simulink model "sim_new_traj_only_att_ctrl"  (R2020a)
settings: Solver=ode4  StartTime=0.0  StopTime=30.0  FixedStep=0.01  RelTol=1e-3
values from neighbouring files (symbols this model uses):
  beta_Phi_1 = pp0 * cal_frac_squ( 3, p_p0_plus_1, q_p0_plus_1 )                          * cal_frac_squ( eps_s_bar / pi, p_p0_min_2, q_p0_min_2 )                          / ( 2 * ( 2 * pp0 - 1 ) * tanh( gamma0 * ( eps_s_bar / pi ) / 2 ) )                          - ( cal_frac_squ( 3, p_p0_plus_1, q_p0_plus_1 ) * gamma0 / ( 4 * ( 2 * pp0 -1 ) ) )                          * cal_frac_squ( eps_s_bar / pi, p_p0_min_ ...(+136 chars)    [init_new_traj_only_att_ctrl.m]
  beta_Phi_2 = ( 1 - pp0 ) * cal_frac_squ( 3, p_p0_plus_1, q_p0_plus_1 )                          / ( 2 * ( 1 - 2 * pp0 ) * cal_frac_squ( eps_s_bar / pi, p_p0_0, q_p0_0 ) * tanh( gamma0 * ( eps_s_bar / pi ) / 2 ) )                          - ( cal_frac_squ( 3, p_p0_plus_1, q_p0_plus_1 ) * gamma0 / ( 4 * ( 1 - 2 * pp0 ) ) )                          * cal_frac_squ( eps_s_bar / pi, p_1_min_p0, q_1_min_p0 )          ...(+112 chars)    [init_new_traj_only_att_ctrl.m]
  c1_diff_sigma_bar_w = diag([12; 12; 12])    [init_new_traj_only_att_ctrl.m]
  c1_diff_ui = diag([25; 30; 20])    [init_new_traj_only_att_ctrl.m]
  c2_diff_sigma_bar_w = diag([12; 12; 12])    [init_new_traj_only_att_ctrl.m]
  c2_diff_ui = diag([50; 50; 10])    [init_new_traj_only_att_ctrl.m]
  c3_diff_sigma_bar_w = diag([15; 15; 15])    [init_new_traj_only_att_ctrl.m]
  c3_diff_ui = diag([15; 15; 10])    [init_new_traj_only_att_ctrl.m]
  c_w_1 = diag( [20; 15; 15] )    [init_new_traj_only_att_ctrl.m]
  c_w_2 = diag( [20; 15; 15] )    [init_new_traj_only_att_ctrl.m]
  c_w_3 = diag( [2; 2; 2] )    [init_new_traj_only_att_ctrl.m]
  cS0 = diag( [4.5; 4.5; 4.5] )    [init_new_traj_only_att_ctrl.m]
  dw_aa_t = 0.2 * ones(3, 5) + ( 1.0 - 0.2 ) * rand(3, 5)    [init_new_traj_only_att_ctrl.m]
  dw_ff_t = [ 0.4 * ones(1, 5) + ( 1.0 - 0.4 ) * rand(1, 5);                      0.4 * ones(1, 5) + ( 1.0 - 0.4 ) * rand(1, 5);                      0.2 * ones(1, 5) + ( 0.6 - 0.2 ) * rand(1, 5) ]    [init_new_traj_only_att_ctrl.m]
  dw_phi_t = ( - pi / 2 ) * ones(3, 5) + ( pi / 2 - ( - pi / 2 ) ) * rand(3, 5)    [init_new_traj_only_att_ctrl.m]
  dwci_init = zeros(3,5)    [init_new_traj_only_att_ctrl.m]
  eps_s_bar_div_pi = eps_s_bar / pi    (= 0.03)    [init_new_traj_only_att_ctrl.m]
  gamma0 = 20    [init_new_traj_only_att_ctrl.m]
  h1w = diag([20.0; 20.0; 20.0])    [init_new_traj_only_att_ctrl.m]
  h2w = diag([30.0; 35.0; 35.0])    [init_new_traj_only_att_ctrl.m]
  h3w = diag([30.0; 25.0; 30.0])    [init_new_traj_only_att_ctrl.m]
  Ji = zeros(3,3,NF)    [init_new_traj_only_att_ctrl.m]
  k_J_0 = diag( [1; 1; 1] )    [init_new_traj_only_att_ctrl.m]
  Lamd_diff_sigma_bar_w = 0.8    [init_new_traj_only_att_ctrl.m]
  Lamd_diff_ui = 0.8    [init_new_traj_only_att_ctrl.m]
  mu_c_theta = 100    [init_new_traj_only_att_ctrl.m]
  mu_d_w = 100    [init_new_traj_only_att_ctrl.m]
  pos0 = zeros(3, 1)    [init_new_traj_only_att_ctrl.m]
  pp0 = 8 / 11    (= 0.727272727273)    [init_new_traj_only_att_ctrl.m]
  PZ0 = P0(3)    [init_new_traj_only_att_ctrl.m]
  PZ1 = 10    [init_new_traj_only_att_ctrl.m]
  Qci_init = repmat([1;0;0;0],1,NF)    [init_new_traj_only_att_ctrl.m]
  R0 = 4    [init_new_traj_only_att_ctrl.m]
  R1 = 8    [init_new_traj_only_att_ctrl.m]
  Rci_init = zeros(3,3,NF)    [init_new_traj_only_att_ctrl.m]
  Ri_init = zeros(3,3,NF)    [init_new_traj_only_att_ctrl.m]
  Rx2 = 10    [init_new_traj_only_att_ctrl.m]
  Ry2 = 6    [init_new_traj_only_att_ctrl.m]
  Rz2 = 4    [init_new_traj_only_att_ctrl.m]
  T0 = 0    [init_new_traj_only_att_ctrl.m]
  T1 = tseq1    (= 10)    [init_new_traj_only_att_ctrl.m]
  T2 = tseq1 + tseq12 + tseq2    (= 30)    [init_new_traj_only_att_ctrl.m]
  thr_p_plus_1 = cal_frac_squ( 3, p_p0_plus_1, q_p0_plus_1 )    [init_new_traj_only_att_ctrl.m]
  ui_init = zeros(3,NF)    [init_new_traj_only_att_ctrl.m]
  vel0 = zeros(3, 1)    [init_new_traj_only_att_ctrl.m]
  wci_init = zeros(3,5)    [init_new_traj_only_att_ctrl.m]
  zeta_diff_sigma_bar_w = 0.3    [init_new_traj_only_att_ctrl.m]
  zeta_diff_ui = 0.05    [init_new_traj_only_att_ctrl.m]
undefined symbols (not defined in the file or in its folder): cal_frac_squ, p_2_p0, p_alfaw1, p_alfaw2, p_beta_w_1, p_beta_w_2, p_p0_min_1, p_p0_plus_1, q_2_p0, q_alfaw1, q_alfaw2, q_beta_w_1, q_beta_w_2, q_p0_min_1, q_p0_plus_1, Qei_init, Qi_init, Rei_init, V_Phi_Rei_init, wei_init, wi_init
(part 4 of 5)

== matlab function sim_new_traj_only_att_ctrl/cal wci dwci agent 5 ==
  data: ui_vec input; wci output; duihat_vec input; d2uihat_vec input; Rci_mat input; dwci output
function [wci, dwci] = fcn(ui_vec, duihat_vec, d2uihat_vec, Rci_mat)
%%%% 计算姿态角速率指令及其导数

iiuav = 5;
ui = ui_vec(:,iiuav);
duihat = duihat_vec(:,iiuav);
d2uihat = d2uihat_vec(:,iiuav);
Rci = Rci_mat(:,:,iiuav);

ee1 = [1;0;0];
ee2 = [0;1;0];
ee3 = [0;0;1];
RciE3 = ui / norm(ui,2);
PiMat = eye(3,3) - ee3*(ee3');
dRciE3 = (1 / norm(ui,2))*Rci*PiMat*(Rci')*duihat;
Themat = [-RciE3(2)/(1+RciE3(3)),         -RciE3(1)/(1+RciE3(3)),       (RciE3(1)*RciE3(2))/((1+RciE3(3))^2); ...
                   2*RciE3(1)/(1+RciE3(3)),                0,                               1 - (RciE3(1)^2)/((1+RciE3(3))^2); ...
                               0                                       -1                                                        0                                   ];
wcxe3 = (1 / norm(ui,2))*PiMat*(Rci')*duihat;
wcxe2 = (1 / norm(ui,2))*(Rci')*Themat*Rci*PiMat*(Rci')*duihat;
wci = [-wcxe3(2); wcxe3(1); -wcxe2(1)];

TempMat1 = [0,                           -1/(1+RciE3(3)),                   (RciE3(2))/((1+RciE3(3))^2); ...
                       2/(1+RciE3(3)),                0,                               (-2*RciE3(1))/((1+RciE3(3))^2); ...
                       0,                                     0,                                                   0                             ];
TempMat2 = [-1/(1+RciE3(3)),              0,                               (RciE3(1))/((1+RciE3(3))^2); ...
                       0,                                     0,                                                   0                      ; ...
                       0,                                     0,                                                   0                             ];
TempMat3 = [(RciE3(2))/((1+RciE3(3))^2),                 (RciE3(1))/((1+RciE3(3))^2),       (-2*RciE3(1)*RciE3(2))/((1+RciE3(3))^3); ...
                       (-2*RciE3(1))/((1+RciE3(3))^2),                             0,                               (2*(RciE3(1)^2))/((1+RciE3(3))^3); ...
                        0,                                                                          0,                                                   0                             ];
dTheMat = TempMat1*dRciE3*(ee1') + TempMat2*dRciE3*(ee2') + TempMat3*dRciE3*(ee3');
wcix = cal_askew_mat(wci);
dRciT = -wcix*(Rci');
dwcxe3 = (1 / norm(ui,2))*PiMat*(dRciT*duihat+(Rci')*(d2uihat-(((ui')*duihat)/(norm(ui,2)^2))*duihat));
dwcxe2 = (1 / norm(ui,2))*((dRciT*Themat+(Rci')*dTheMat) ...
                *(Rci*PiMat*(Rci'))*duihat + (Rci')*Themat*(Rci*PiMat*(Rci'))*(d2uihat-(((ui')*duihat)/(norm(ui,2)^2))*duihat));
dwci = [-dwcxe3(2);  dwcxe3(1);  -dwcxe2(1)];

== matlab function sim_new_traj_only_att_ctrl/cal wei agent 1 ==
  data: wi_vec input; wei_1 output; Rei_vec input; wci_vec input
function wei_1 = fcn(wi_vec, Rei_vec, wci_vec)
%%%% 更新姿态角速率误差
iiuav = 1;
wei_1 = wi_vec(:,iiuav) - (Rei_vec(:,:,iiuav)') * wci_vec(:,iiuav);

end

== matlab function sim_new_traj_only_att_ctrl/cal wei agent 2 ==
  data: wi_vec input; wei_2 output; Rei_vec input; wci_vec input
function wei_2 = fcn(wi_vec, Rei_vec, wci_vec)
%%%% 更新姿态角速率误差
iiuav = 2;
wei_2 = wi_vec(:,iiuav) - (Rei_vec(:,:,iiuav)') * wci_vec(:,iiuav);

end

== matlab function sim_new_traj_only_att_ctrl/cal wei agent 3 ==
  data: wi_vec input; wei_3 output; Rei_vec input; wci_vec input
function wei_3 = fcn(wi_vec, Rei_vec, wci_vec)
%%%% 更新姿态角速率误差
iiuav = 3;
wei_3 = wi_vec(:,iiuav) - (Rei_vec(:,:,iiuav)') * wci_vec(:,iiuav);

end

== matlab function sim_new_traj_only_att_ctrl/cal wei agent 4 ==
  data: wi_vec input; wei_4 output; Rei_vec input; wci_vec input
function wei_4 = fcn(wi_vec, Rei_vec, wci_vec)
%%%% 更新姿态角速率误差
iiuav = 4;
wei_4 = wi_vec(:,iiuav) - (Rei_vec(:,:,iiuav)') * wci_vec(:,iiuav);

end

== matlab function sim_new_traj_only_att_ctrl/cal wei agent 5 ==
  data: wi_vec input; wei_5 output; Rei_vec input; wci_vec input
function wei_5 = fcn(wi_vec, Rei_vec, wci_vec)
%%%% 更新姿态角速率误差
iiuav = 5;
wei_5 = wi_vec(:,iiuav) - (Rei_vec(:,:,iiuav)') * wci_vec(:,iiuav);

end

== matlab function sim_new_traj_only_att_ctrl/choose ksi_est_err 41 ==
  data: x input; y output
function y = fcn(x)
iiuav = 1;
y = x(:,iiuav);

== matlab function sim_new_traj_only_att_ctrl/choose ksi_est_err 42 ==
  data: x input; y output
function y = fcn(x)
iiuav = 5;
y = x(:,iiuav);

== matlab function sim_new_traj_only_att_ctrl/choose ksi_est_err 43 ==
  data: x input; y output
function y = fcn(x)
iiuav = 1;
y = x(:,iiuav);

== matlab function sim_new_traj_only_att_ctrl/choose ksi_est_err 44 ==
  data: x input; y output
function y = fcn(x)
iiuav = 1;
y = x(:,iiuav);

== matlab function sim_new_traj_only_att_ctrl/choose ksi_est_err 45 ==
  data: x input; y output
function y = fcn(x)
iiuav = 2;
y = x(:,iiuav);

== matlab function sim_new_traj_only_att_ctrl/choose ksi_est_err 46 ==
  data: x input; y output
function y = fcn(x)
iiuav = 2;
y = x(:,iiuav);

== matlab function sim_new_traj_only_att_ctrl/choose ksi_est_err 47 ==
  data: x input; y output
function y = fcn(x)
iiuav = 3;
y = x(:,iiuav);

== matlab function sim_new_traj_only_att_ctrl/choose ksi_est_err 48 ==
  data: x input; y output
function y = fcn(x)
iiuav = 3;
y = x(:,iiuav);

== matlab function sim_new_traj_only_att_ctrl/choose ksi_est_err 49 ==
  data: x input; y output
function y = fcn(x)
iiuav = 4;
y = x(:,iiuav);

== matlab function sim_new_traj_only_att_ctrl/cal Fi_S agent 4 ==
  data: cS0 input; Ji input; wi_vec input; wci_vec input; wei_vec input; Fi_S_4 output; dwci_vec input; Rei_vec input; Phi_bar_psi_e_vec input
function Fi_S_4 = fcn(cS0, Ji, wi_vec, wci_vec, wei_vec, dwci_vec, Rei_vec, Phi_bar_psi_e_vec)
%%%% 计算补偿项
iiuav = 4;
Fi_S_4 = -cal_askew_mat( wi_vec(:,iiuav) ) * Ji(:,:,iiuav) * wi_vec(:,iiuav) ...
                + Ji(:,:,iiuav) * cal_askew_mat( wei_vec(:,iiuav) ) * ( Rei_vec(:,:,iiuav)' ) * wci_vec(:,iiuav) ...
                - Ji(:,:,iiuav) * ( Rei_vec(:,:,iiuav)' ) * dwci_vec(:,iiuav) ...
                + cS0 * Ji(:,:,iiuav) * Phi_bar_psi_e_vec(:,iiuav);

== matlab function sim_new_traj_only_att_ctrl/choose ksi_est_err 50 ==
  data: x input; y output
function y = fcn(x)
iiuav = 4;
y = x(:,iiuav);

== matlab function sim_new_traj_only_att_ctrl/choose ksi_est_err 51 ==
  data: x input; y output
function y = fcn(x)
iiuav = 5;
y = x(:,iiuav);

== matlab function sim_new_traj_only_att_ctrl/choose ksi_est_err 52 ==
  data: x input; y output
function y = fcn(x)
iiuav = 1;
y = x(:,iiuav);

== matlab function sim_new_traj_only_att_ctrl/choose ksi_est_err 53 ==
  data: x input; y output
function y = fcn(x)
iiuav = 5;
y = x(:,iiuav);

== matlab function sim_new_traj_only_att_ctrl/choose ksi_est_err 54 ==
  data: x input; y output
function y = fcn(x)
iiuav = 1;
y = x(:,iiuav);

== matlab function sim_new_traj_only_att_ctrl/choose ksi_est_err 55 ==
  data: x input; y output
function y = fcn(x)
iiuav = 2;
y = x(:,iiuav);

== matlab function sim_new_traj_only_att_ctrl/choose ksi_est_err 56 ==
  data: x input; y output
function y = fcn(x)
iiuav = 3;
y = x(:,iiuav);

== matlab function sim_new_traj_only_att_ctrl/choose ksi_est_err 57 ==
  data: x input; y output
function y = fcn(x)
iiuav = 4;
y = x(:,iiuav);

== matlab function sim_new_traj_only_att_ctrl/choose ksi_est_err 58 ==
  data: x input; y output
function y = fcn(x)
iiuav = 5;
y = x(:,iiuav);

== matlab function sim_new_traj_only_att_ctrl/choose ksi_est_err 59 ==
  data: x input; y output
function y = fcn(x)
iiuav = 1;
y = x(:,iiuav);

== matlab function sim_new_traj_only_att_ctrl/choose ksi_est_err 60 ==
  data: x input; y output
function y = fcn(x)
iiuav = 1;
y = x(:,iiuav);

== matlab function sim_new_traj_only_att_ctrl/choose ksi_est_err 61 ==
  data: x input; y output
function y = fcn(x)
iiuav = 2;
y = x(:,iiuav);

== matlab function sim_new_traj_only_att_ctrl/choose ksi_est_err 62 ==
  data: x input; y output
function y = fcn(x)
iiuav = 2;
y = x(:,iiuav);

== matlab function sim_new_traj_only_att_ctrl/choose ksi_est_err 63 ==
  data: x input; y output
function y = fcn(x)
iiuav = 2;
y = x(:,iiuav);

== matlab function sim_new_traj_only_att_ctrl/choose ksi_est_err 64 ==
  data: x input; y output
function y = fcn(x)
iiuav = 3;
y = x(:,iiuav);

== matlab function sim_new_traj_only_att_ctrl/choose ksi_est_err 65 ==
  data: x input; y output
function y = fcn(x)
iiuav = 3;
y = x(:,iiuav);

== matlab function sim_new_traj_only_att_ctrl/choose ksi_est_err 66 ==
  data: x input; y output
function y = fcn(x)
iiuav = 4;
y = x(:,iiuav);

== matlab function sim_new_traj_only_att_ctrl/choose ksi_est_err 67 ==
  data: x input; y output
function y = fcn(x)
iiuav = 4;
y = x(:,iiuav);

== matlab function sim_new_traj_only_att_ctrl/choose ksi_est_err 68 ==
  data: x input; y output
function y = fcn(x)
iiuav = 5;
y = x(:,iiuav);

== matlab function sim_new_traj_only_att_ctrl/choose ksi_est_err 69 ==
  data: x input; y output
function y = fcn(x)
iiuav = 5;
y = x(:,iiuav);

== matlab function sim_new_traj_only_att_ctrl/cal Fi_S agent 5 ==
  data: cS0 input; Ji input; wi_vec input; wci_vec input; wei_vec input; Fi_S_5 output; dwci_vec input; Rei_vec input; Phi_bar_psi_e_vec input
function Fi_S_5 = fcn(cS0, Ji, wi_vec, wci_vec, wei_vec, dwci_vec, Rei_vec, Phi_bar_psi_e_vec)
%%%% 计算补偿项
iiuav = 5;
Fi_S_5 = -cal_askew_mat( wi_vec(:,iiuav) ) * Ji(:,:,iiuav) * wi_vec(:,iiuav) ...
                + Ji(:,:,iiuav) * cal_askew_mat( wei_vec(:,iiuav) ) * ( Rei_vec(:,:,iiuav)' ) * wci_vec(:,iiuav) ...
                - Ji(:,:,iiuav) * ( Rei_vec(:,:,iiuav)' ) * dwci_vec(:,iiuav) ...
                + cS0 * Ji(:,:,iiuav) * Phi_bar_psi_e_vec(:,iiuav);

== matlab function sim_new_traj_only_att_ctrl/choose ksi_est_err 70 ==
  data: x input; y output
function y = fcn(x)
iiuav = 2;
y = x(:,iiuav);

== matlab function sim_new_traj_only_att_ctrl/choose ksi_est_err 71 ==
  data: x input; y output
function y = fcn(x)
iiuav = 3;
y = x(:,iiuav);

== matlab function sim_new_traj_only_att_ctrl/choose ksi_est_err 72 ==
  data: x input; y output
function y = fcn(x)
iiuav = 3;
y = x(:,iiuav);

== matlab function sim_new_traj_only_att_ctrl/choose ksi_est_err 73 ==
  data: x input; y output
function y = fcn(x)
iiuav = 4;
y = x(:,iiuav);

== matlab function sim_new_traj_only_att_ctrl/choose ksi_est_err 74 ==
  data: x input; y output
function y = fcn(x)
iiuav = 4;
y = x(:,iiuav);

== matlab function sim_new_traj_only_att_ctrl/choose ksi_est_err 75 ==
  data: x input; y output
function y = fcn(x)
iiuav = 5;
y = x(:,iiuav);

== matlab function sim_new_traj_only_att_ctrl/choose ui agent 1 ==
  data: x input; y output
function y = fcn(x)
iiuav = 1;
y = x(:,iiuav);

== matlab function sim_new_traj_only_att_ctrl/choose ui agent 2 ==
  data: x input; y output
function y = fcn(x)
iiuav = 2;
y = x(:,iiuav);

== matlab function sim_new_traj_only_att_ctrl/choose ui agent 3 ==
  data: x input; y output
function y = fcn(x)
iiuav = 3;
y = x(:,iiuav);

== matlab function sim_new_traj_only_att_ctrl/choose ui agent 4 ==
  data: x input; y output
function y = fcn(x)
iiuav = 4;
y = x(:,iiuav);

== matlab function sim_new_traj_only_att_ctrl/choose ui agent 5 ==
  data: x input; y output
function y = fcn(x)
iiuav = 5;
y = x(:,iiuav);

== matlab function sim_new_traj_only_att_ctrl/combine Fi_S ==
  data: Fi_S_1 input; Fi_S_2 input; Fi_S_3 input; Fi_S_4 input; Fi_S_5 input; Fi_S_vec output
function Fi_S_vec  = fcn(Fi_S_1, Fi_S_2, Fi_S_3, Fi_S_4, Fi_S_5)
%%%% 合并补偿项
Fi_S_vec = zeros(3,5);
Fi_S_vec(:,1) = Fi_S_1(:);
Fi_S_vec(:,2) = Fi_S_2(:);
Fi_S_vec(:,3) = Fi_S_3(:);
Fi_S_vec(:,4) = Fi_S_4(:);
Fi_S_vec(:,5) = Fi_S_5(:);

== matlab function sim_new_traj_only_att_ctrl/combine Phi_bar_psi_e ==
  data: Phi_bar_psi_e_node_1 input; Phi_bar_psi_e_node_2 input; Phi_bar_psi_e_node_3 input; Phi_bar_psi_e_node_4 input; Phi_bar_psi_e_node_5 input; Phi_bar_psi_e_vec output
function Phi_bar_psi_e_vec  = fcn(Phi_bar_psi_e_node_1, Phi_bar_psi_e_node_2, Phi_bar_psi_e_node_3, ...
                                                                Phi_bar_psi_e_node_4, Phi_bar_psi_e_node_5)
%%%% 合并姿态误差导数
Phi_bar_psi_e_vec = zeros(3,5);
Phi_bar_psi_e_vec(:,1) = Phi_bar_psi_e_node_1(:);
Phi_bar_psi_e_vec(:,2) = Phi_bar_psi_e_node_2(:);
Phi_bar_psi_e_vec(:,3) = Phi_bar_psi_e_node_3(:);
Phi_bar_psi_e_vec(:,4) = Phi_bar_psi_e_node_4(:);
Phi_bar_psi_e_vec(:,5) = Phi_bar_psi_e_node_5(:);

== matlab function sim_new_traj_only_att_ctrl/combine Phi_psi_e ==
  data: Phi_psi_e_node_1 input; Phi_psi_e_node_2 input; Phi_psi_e_node_3 input; Phi_psi_e_node_4 input; Phi_psi_e_node_5 input; Phi_psi_e_vec output
function Phi_psi_e_vec  = fcn(Phi_psi_e_node_1, Phi_psi_e_node_2, Phi_psi_e_node_3, ...
                                                        Phi_psi_e_node_4, Phi_psi_e_node_5)
%%%% 合并姿态误差项
Phi_psi_e_vec = zeros(3,5);
Phi_psi_e_vec(:,1) = Phi_psi_e_node_1(:);
Phi_psi_e_vec(:,2) = Phi_psi_e_node_2(:);
Phi_psi_e_vec(:,3) = Phi_psi_e_node_3(:);
Phi_psi_e_vec(:,4) = Phi_psi_e_node_4(:);
Phi_psi_e_vec(:,5) = Phi_psi_e_node_5(:);

== matlab function sim_new_traj_only_att_ctrl/combine Qci Rci ==
  data: Qci_1 input; Qci_vec output; Qci_2 input; Qci_3 input; Qci_4 input; Qci_5 input; Rci_1 input; Rci_2 input; Rci_3 input; Rci_4 input; Rci_5 input; Rci_vec output
function [Qci_vec, Rci_vec] = fcn(Qci_1, Qci_2, Qci_3, Qci_4, Qci_5, ...
                                                            Rci_1, Rci_2, Rci_3, Rci_4, Rci_5)
%%%% 合并四元数和姿态旋转矩阵
Qci_vec = zeros(4,5);
Qci_vec(:,1) = Qci_1(:);
Qci_vec(:,2) = Qci_2(:);
Qci_vec(:,3) = Qci_3(:);
Qci_vec(:,4) = Qci_4(:);
Qci_vec(:,5) = Qci_5(:);

Rci_vec = zeros(3,3,5);
Rci_vec(:,:,1) = Rci_1;
Rci_vec(:,:,2) = Rci_2;
Rci_vec(:,:,3) = Rci_3;
Rci_vec(:,:,4) = Rci_4;
Rci_vec(:,:,5) = Rci_5;

== matlab function sim_new_traj_only_att_ctrl/combine Qci Rci1 ==
  data: V_Phi_Rei_1 input; V_Phi_Rei_vec output; V_Phi_Rei_2 input; V_Phi_Rei_3 input; V_Phi_Rei_4 input; V_Phi_Rei_5 input
function V_Phi_Rei_vec = fcn(V_Phi_Rei_1, V_Phi_Rei_2, V_Phi_Rei_3, V_Phi_Rei_4, V_Phi_Rei_5)
%%%% 合并LogSO3空间的辅助姿态误差向量
V_Phi_Rei_vec = [V_Phi_Rei_1(:), V_Phi_Rei_2(:), V_Phi_Rei_3(:), V_Phi_Rei_4(:), V_Phi_Rei_5(:)];

== matlab function sim_new_traj_only_att_ctrl/cal Phi_bar_psi_e agent 1 ==
  data: pp0 input; Phi_bar_psi_e_node_1 output; beta_Phi_1 input; beta_Phi_2 input; thr_p_plus_1 input; gamma0 input; eps_s_bar_div_pi input; wei_vec input; S_bar_vec input; V_Phi_Rei_div_pi_vec input; V_Phi_Rei_squ_p_min_1_vec input; V_Phi_Rei_squ_p_plus_1_vec input; V_Phi_Rei_squ_2p_vec input
function Phi_bar_psi_e_node_1 = fcn(pp0, beta_Phi_1, beta_Phi_2, thr_p_plus_1, gamma0, ...
                                                                    eps_s_bar_div_pi, wei_vec, S_bar_vec, V_Phi_Rei_div_pi_vec, ...
                                                                    V_Phi_Rei_squ_p_min_1_vec, V_Phi_Rei_squ_p_plus_1_vec, V_Phi_Rei_squ_2p_vec)
%%%% 计算姿态误差项
iiuav = 1;
Phi_bar_psi_e_node_1 = zeros(3,1);
for kk = 1:3
    if S_bar_vec(kk, iiuav) == 0
        Phi_bar_psi_e_node_1(kk, 1) = thr_p_plus_1 * ( pp0 + 1 ) * V_Phi_Rei_div_pi_vec(kk, iiuav) ...
                                                                * V_Phi_Rei_squ_p_min_1_vec(kk, iiuav) * wei_vec(kk, iiuav) ...
                                                                / ( 2 * tanh( ( gamma0 / 2 ) * V_Phi_Rei_div_pi_vec(kk, iiuav) ) ) ...
                                                                + ( thr_p_plus_1 * gamma0 / 4 ) * V_Phi_Rei_squ_p_plus_1_vec(kk, iiuav) ...
                                                                * ( ( sech( ( gamma0 / 2 ) * V_Phi_Rei_div_pi_vec(kk, iiuav) ) ...
                                                                / tanh( ( gamma0 / 2 ) * V_Phi_Rei_div_pi_vec(kk, iiuav) ) ) ^ 2 ) * wei_vec(kk, iiuav);
    else
        if abs( V_Phi_Rei_div_pi_vec ) > eps_s_bar_div_pi
            Phi_bar_psi_e_node_1(kk, 1) = thr_p_plus_1 * ( pp0 + 1 ) * V_Phi_Rei_div_pi_vec(kk, iiuav) ...
                                                                    * V_Phi_Rei_squ_p_min_1_vec(kk, iiuav) * wei_vec(kk, iiuav) ...
                                                                    / ( 2 * tanh( ( gamma0 / 2 ) * V_Phi_Rei_div_pi_vec(kk, iiuav) ) ) ...
                                                                    + ( thr_p_plus_1 * gamma0 / 4 ) * V_Phi_Rei_squ_p_plus_1_vec(kk, iiuav) ...
                                                                    * ( ( sech( ( gamma0 / 2 ) * V_Phi_Rei_div_pi_vec(kk, iiuav) ) ...
                                                                    / tanh( ( gamma0 / 2 ) * V_Phi_Rei_div_pi_vec(kk, iiuav) ) ) ^ 2 ) * wei_vec(kk, iiuav);
        else
            Phi_bar_psi_e_node_1(kk, 1) = 2 * beta_Phi_1 * ( ( abs( V_Phi_Rei_div_pi_vec(kk, iiuav) ) ) ^ 2 ) * wei_vec(kk, iiuav) ...
                                                                    + ( 2 * pp0 + 1 ) * beta_Phi_2 * V_Phi_Rei_squ_2p_vec(kk, iiuav) * wei_vec(kk, iiuav);
        end
    end
end

== matlab function sim_new_traj_only_att_ctrl/combine Qi Ri ==
  data: Qi_1 input; Qi_vec output; Qi_2 input; Qi_3 input; Qi_4 input; Qi_5 input; Ri_1 input; Ri_2 input; Ri_3 input; Ri_4 input; Ri_5 input; Ri_vec output
function [Qi_vec, Ri_vec] = fcn(Qi_1, Qi_2, Qi_3, Qi_4, Qi_5, ...
                                                        Ri_1, Ri_2, Ri_3, Ri_4, Ri_5)
%%%% 合并四元数和姿态旋转矩阵
Qi_vec = zeros(4,5);
Qi_vec(:,1) = Qi_1(:);
Qi_vec(:,2) = Qi_2(:);
Qi_vec(:,3) = Qi_3(:);
Qi_vec(:,4) = Qi_4(:);
Qi_vec(:,5) = Qi_5(:);

Ri_vec = zeros(3,3,5);
Ri_vec(:,:,1) = Ri_1;
Ri_vec(:,:,2) = Ri_2;
Ri_vec(:,:,3) = Ri_3;
Ri_vec(:,:,4) = Ri_4;
Ri_vec(:,:,5) = Ri_5;

== matlab function sim_new_traj_only_att_ctrl/combine S_bar ==
  data: S_bar_node_1 input; S_bar_node_2 input; S_bar_node_3 input; S_bar_node_4 input; S_bar_node_5 input; S_bar_vec output
function S_bar_vec  = fcn(S_bar_node_1, S_bar_node_2, S_bar_node_3, ...
                                                S_bar_node_4, S_bar_node_5)
%%%% 合并辅助滑模面
S_bar_vec = zeros(3,5);
S_bar_vec(:,1) = S_bar_node_1(:);
S_bar_vec(:,2) = S_bar_node_2(:);
S_bar_vec(:,3) = S_bar_node_3(:);
S_bar_vec(:,4) = S_bar_node_4(:);
S_bar_vec(:,5) = S_bar_node_5(:);

== matlab function sim_new_traj_only_att_ctrl/combine Si ==
  data: Si_1 input; Si_2 input; Si_3 input; Si_4 input; Si_5 input; Si_vec output
function Si_vec  = fcn(Si_1, Si_2, Si_3, Si_4, Si_5)
%%%% 合并滑模面
Si_vec = zeros(3,5);
Si_vec(:,1) = Si_1(:);
Si_vec(:,2) = Si_2(:);
Si_vec(:,3) = Si_3(:);
Si_vec(:,4) = Si_4(:);
Si_vec(:,5) = Si_5(:);

== matlab function sim_new_traj_only_att_ctrl/combine Si_squ_beta_w_1 ==
  data: Si_squ_beta_w_1_node_1 input; Si_squ_beta_w_1_node_2 input; Si_squ_beta_w_1_node_3 input; Si_squ_beta_w_1_node_4 input; Si_squ_beta_w_1_node_5 input; Si_squ_beta_w_1_vec output
function Si_squ_beta_w_1_vec  = fcn(Si_squ_beta_w_1_node_1, Si_squ_beta_w_1_node_2, Si_squ_beta_w_1_node_3, ...
                                                                    Si_squ_beta_w_1_node_4, Si_squ_beta_w_1_node_5)
%%%% 合并误差幂次项
Si_squ_beta_w_1_vec = zeros(3,5);
Si_squ_beta_w_1_vec(:,1) = Si_squ_beta_w_1_node_1(:);
Si_squ_beta_w_1_vec(:,2) = Si_squ_beta_w_1_node_2(:);
Si_squ_beta_w_1_vec(:,3) = Si_squ_beta_w_1_node_3(:);
Si_squ_beta_w_1_vec(:,4) = Si_squ_beta_w_1_node_4(:);
Si_squ_beta_w_1_vec(:,5) = Si_squ_beta_w_1_node_5(:);

== matlab function sim_new_traj_only_att_ctrl/combine Si_squ_beta_w_2 ==
  data: Si_squ_beta_w_2_node_1 input; Si_squ_beta_w_2_node_2 input; Si_squ_beta_w_2_node_3 input; Si_squ_beta_w_2_node_4 input; Si_squ_beta_w_2_node_5 input; Si_squ_beta_w_2_vec output
function Si_squ_beta_w_2_vec  = fcn(Si_squ_beta_w_2_node_1, Si_squ_beta_w_2_node_2, Si_squ_beta_w_2_node_3, ...
                                                                    Si_squ_beta_w_2_node_4, Si_squ_beta_w_2_node_5)
%%%% 合并误差幂次项
Si_squ_beta_w_2_vec = zeros(3,5);
Si_squ_beta_w_2_vec(:,1) = Si_squ_beta_w_2_node_1(:);
Si_squ_beta_w_2_vec(:,2) = Si_squ_beta_w_2_node_2(:);
Si_squ_beta_w_2_vec(:,3) = Si_squ_beta_w_2_node_3(:);
Si_squ_beta_w_2_vec(:,4) = Si_squ_beta_w_2_node_4(:);
Si_squ_beta_w_2_vec(:,5) = Si_squ_beta_w_2_node_5(:);

== matlab function sim_new_traj_only_att_ctrl/combine V_Phi_Rei_squ_2p ==
  data: V_Phi_Rei_squ_2p_node_1 input; V_Phi_Rei_squ_2p_node_2 input; V_Phi_Rei_squ_2p_node_3 input; V_Phi_Rei_squ_2p_node_4 input; V_Phi_Rei_squ_2p_node_5 input; V_Phi_Rei_squ_2p_vec output
function V_Phi_Rei_squ_2p_vec  = fcn(V_Phi_Rei_squ_2p_node_1, V_Phi_Rei_squ_2p_node_2, V_Phi_Rei_squ_2p_node_3, ...
                                                                        V_Phi_Rei_squ_2p_node_4, V_Phi_Rei_squ_2p_node_5)
%%%% 合并姿态误差指数坐标
V_Phi_Rei_squ_2p_vec = zeros(3,5);
V_Phi_Rei_squ_2p_vec(:,1) = V_Phi_Rei_squ_2p_node_1(:);
V_Phi_Rei_squ_2p_vec(:,2) = V_Phi_Rei_squ_2p_node_2(:);
V_Phi_Rei_squ_2p_vec(:,3) = V_Phi_Rei_squ_2p_node_3(:);
V_Phi_Rei_squ_2p_vec(:,4) = V_Phi_Rei_squ_2p_node_4(:);
V_Phi_Rei_squ_2p_vec(:,5) = V_Phi_Rei_squ_2p_node_5(:);

== matlab function sim_new_traj_only_att_ctrl/combine V_Phi_Rei_squ_p_min_1 ==
  data: V_Phi_Rei_squ_p_min_1_node_1 input; V_Phi_Rei_squ_p_min_1_node_2 input; V_Phi_Rei_squ_p_min_1_node_3 input; V_Phi_Rei_squ_p_min_1_node_4 input; V_Phi_Rei_squ_p_min_1_node_5 input; V_Phi_Rei_squ_p_min_1_vec output
function V_Phi_Rei_squ_p_min_1_vec  = fcn(V_Phi_Rei_squ_p_min_1_node_1, V_Phi_Rei_squ_p_min_1_node_2, V_Phi_Rei_squ_p_min_1_node_3, ...
                                                                                V_Phi_Rei_squ_p_min_1_node_4, V_Phi_Rei_squ_p_min_1_node_5)
%%%% 合并姿态误差导数
V_Phi_Rei_squ_p_min_1_vec = zeros(3,5);
V_Phi_Rei_squ_p_min_1_vec(:,1) = V_Phi_Rei_squ_p_min_1_node_1(:);
V_Phi_Rei_squ_p_min_1_vec(:,2) = V_Phi_Rei_squ_p_min_1_node_2(:);
V_Phi_Rei_squ_p_min_1_vec(:,3) = V_Phi_Rei_squ_p_min_1_node_3(:);
V_Phi_Rei_squ_p_min_1_vec(:,4) = V_Phi_Rei_squ_p_min_1_node_4(:);
V_Phi_Rei_squ_p_min_1_vec(:,5) = V_Phi_Rei_squ_p_min_1_node_5(:);

== matlab function sim_new_traj_only_att_ctrl/combine V_Phi_Rei_squ_p_plus_1 ==
  data: V_Phi_Rei_squ_p_plus_1_node_1 input; V_Phi_Rei_squ_p_plus_1_node_2 input; V_Phi_Rei_squ_p_plus_1_node_3 input; V_Phi_Rei_squ_p_plus_1_node_4 input; V_Phi_Rei_squ_p_plus_1_node_5 input; V_Phi_Rei_squ_p_plus_1_vec output
function V_Phi_Rei_squ_p_plus_1_vec  = fcn(V_Phi_Rei_squ_p_plus_1_node_1, V_Phi_Rei_squ_p_plus_1_node_2, V_Phi_Rei_squ_p_plus_1_node_3, ...
                                                                                V_Phi_Rei_squ_p_plus_1_node_4, V_Phi_Rei_squ_p_plus_1_node_5)
%%%% 合并姿态误差指数坐标
V_Phi_Rei_squ_p_plus_1_vec = zeros(3,5);
V_Phi_Rei_squ_p_plus_1_vec(:,1) = V_Phi_Rei_squ_p_plus_1_node_1(:);
V_Phi_Rei_squ_p_plus_1_vec(:,2) = V_Phi_Rei_squ_p_plus_1_node_2(:);
V_Phi_Rei_squ_p_plus_1_vec(:,3) = V_Phi_Rei_squ_p_plus_1_node_3(:);
V_Phi_Rei_squ_p_plus_1_vec(:,4) = V_Phi_Rei_squ_p_plus_1_node_4(:);
V_Phi_Rei_squ_p_plus_1_vec(:,5) = V_Phi_Rei_squ_p_plus_1_node_5(:);

== matlab function sim_new_traj_only_att_ctrl/combine d_sigma_bar_v_est1 ==
  data: d_sigma_bar_w_est_1 input; d_sigma_bar_w_est_2 input; d_sigma_bar_w_est_3 input; d_sigma_bar_w_est_4 input; d_sigma_bar_w_est_5 input; d_sigma_bar_w_vec output
function d_sigma_bar_w_vec  = fcn(d_sigma_bar_w_est_1, d_sigma_bar_w_est_2, d_sigma_bar_w_est_3, d_sigma_bar_w_est_4, d_sigma_bar_w_est_5)
%%%% 合并用微分器求得的虚拟速度控制量导数
d_sigma_bar_w_vec = [d_sigma_bar_w_est_1(:), d_sigma_bar_w_est_2(:), d_sigma_bar_w_est_3(:), d_sigma_bar_w_est_4(:), d_sigma_bar_w_est_5(:)];

== matlab function sim_new_traj_only_att_ctrl/combine duihat d2uihat ==
  data: d_ui_hat_node_1 input; duihat_vec output; d2uihat_vec output; d_ui_hat_node_2 input; d_ui_hat_node_3 input; d_ui_hat_node_4 input; d_ui_hat_node_5 input; d2_ui_hat_node_1 input; d2_ui_hat_node_2 input; d2_ui_hat_node_3 input; d2_ui_hat_node_4 input; d2_ui_hat_node_5 input
function [duihat_vec, d2uihat_vec] = fcn(d_ui_hat_node_1, d_ui_hat_node_2, d_ui_hat_node_3, d_ui_hat_node_4, d_ui_hat_node_5, ...
                                                                            d2_ui_hat_node_1, d2_ui_hat_node_2, d2_ui_hat_node_3, d2_ui_hat_node_4, d2_ui_hat_node_5)

duihat_vec = [d_ui_hat_node_1(:), d_ui_hat_node_2(:), d_ui_hat_node_3(:), d_ui_hat_node_4(:), d_ui_hat_node_5(:)];
d2uihat_vec = [d2_ui_hat_node_1(:), d2_ui_hat_node_2(:), d2_ui_hat_node_3(:), d2_ui_hat_node_4(:), d2_ui_hat_node_5(:)];

== matlab function sim_new_traj_only_att_ctrl/combine dw_hat ==
  data: dw_hat_1 input; dw_hat_2 input; dw_hat_3 input; dw_hat_4 input; dw_hat_5 input; dw_hat_vec output
function dw_hat_vec  = fcn(dw_hat_1, dw_hat_2, dw_hat_3, dw_hat_4, dw_hat_5)
%%%% 合并扰动观测值dw_hat
dw_hat_vec = [dw_hat_1(:), dw_hat_2(:), dw_hat_3(:), dw_hat_4(:), dw_hat_5(:)];

== matlab function sim_new_traj_only_att_ctrl/combine dwi ==
  data: wi_1 input; wi_vec output; wi_2 input; wi_3 input; wi_4 input; wi_5 input
function wi_vec = fcn(wi_1, wi_2, wi_3, wi_4, wi_5)
%%%% 合并姿态角速率
wi_vec = [wi_1(:), wi_2(:), wi_3(:), wi_4(:), wi_5(:)];

== matlab function sim_new_traj_only_att_ctrl/combine sigma_bar_w_hat ==
  data: sigma_bar_w_hat_1 input; sigma_bar_w_hat_2 input; sigma_bar_w_hat_3 input; sigma_bar_w_hat_4 input; sigma_bar_w_hat_5 input; sigma_bar_w_hat_vec output
function sigma_bar_w_hat_vec  = fcn(sigma_bar_w_hat_1, sigma_bar_w_hat_2, sigma_bar_w_hat_3, sigma_bar_w_hat_4, sigma_bar_w_hat_5)
%%%% 合并虚拟速度控制量观测值sigma_bar_w_hat
sigma_bar_w_hat_vec = [sigma_bar_w_hat_1(:), sigma_bar_w_hat_2(:), sigma_bar_w_hat_3(:), sigma_bar_w_hat_4(:), sigma_bar_w_hat_5(:)];

== matlab function sim_new_traj_only_att_ctrl/combine sigma_w ==
  data: sigma_w_1 input; sigma_w_vec output; sigma_w_2 input; sigma_w_3 input; sigma_w_4 input; sigma_w_5 input
function sigma_w_vec = fcn(sigma_w_1, sigma_w_2, sigma_w_3, sigma_w_4, sigma_w_5)
%%%% 合并辅助姿态角速率
sigma_w_vec = [sigma_w_1(:), sigma_w_2(:), sigma_w_3(:), sigma_w_4(:), sigma_w_5(:)];

== matlab function sim_new_traj_only_att_ctrl/combine tau ==
  data: tau_1 input; taui_vec output; tau_2 input; tau_3 input; tau_4 input; tau_5 input
function taui_vec = fcn(tau_1, tau_2, tau_3, tau_4, tau_5)
%%%% 合并辅助姿态角速率
taui_vec = [tau_1(:), tau_2(:), tau_3(:), tau_4(:), tau_5(:)];

== matlab function sim_new_traj_only_att_ctrl/cal Phi_bar_psi_e agent 2 ==
  data: pp0 input; Phi_bar_psi_e_node_2 output; beta_Phi_1 input; beta_Phi_2 input; thr_p_plus_1 input; gamma0 input; eps_s_bar_div_pi input; wei_vec input; S_bar_vec input; V_Phi_Rei_div_pi_vec input; V_Phi_Rei_squ_p_min_1_vec input; V_Phi_Rei_squ_p_plus_1_vec input; V_Phi_Rei_squ_2p_vec input
function Phi_bar_psi_e_node_2 = fcn(pp0, beta_Phi_1, beta_Phi_2, thr_p_plus_1, gamma0, ...
                                                                    eps_s_bar_div_pi, wei_vec, S_bar_vec, V_Phi_Rei_div_pi_vec, ...
                                                                    V_Phi_Rei_squ_p_min_1_vec, V_Phi_Rei_squ_p_plus_1_vec, V_Phi_Rei_squ_2p_vec)
%%%% 计算姿态误差项
iiuav = 2;
Phi_bar_psi_e_node_2 = zeros(3,1);
for kk = 1:3
    if S_bar_vec(kk, iiuav) == 0
        Phi_bar_psi_e_node_2(kk, 1) = thr_p_plus_1 * ( pp0 + 1 ) * V_Phi_Rei_div_pi_vec(kk, iiuav) ...
                                                                * V_Phi_Rei_squ_p_min_1_vec(kk, iiuav) * wei_vec(kk, iiuav) ...
                                                                / ( 2 * tanh( ( gamma0 / 2 ) * V_Phi_Rei_div_pi_vec(kk, iiuav) ) ) ...
                                                                + ( thr_p_plus_1 * gamma0 / 4 ) * V_Phi_Rei_squ_p_plus_1_vec(kk, iiuav) ...
                                                                * ( ( sech( ( gamma0 / 2 ) * V_Phi_Rei_div_pi_vec(kk, iiuav) ) ...
                                                                / tanh( ( gamma0 / 2 ) * V_Phi_Rei_div_pi_vec(kk, iiuav) ) ) ^ 2 ) * wei_vec(kk, iiuav);
    else
        if abs( V_Phi_Rei_div_pi_vec ) > eps_s_bar_div_pi
            Phi_bar_psi_e_node_2(kk, 1) = thr_p_plus_1 * ( pp0 + 1 ) * V_Phi_Rei_div_pi_vec(kk, iiuav) ...
                                                                    * V_Phi_Rei_squ_p_min_1_vec(kk, iiuav) * wei_vec(kk, iiuav) ...
                                                                    / ( 2 * tanh( ( gamma0 / 2 ) * V_Phi_Rei_div_pi_vec(kk, iiuav) ) ) ...
                                                                    + ( thr_p_plus_1 * gamma0 / 4 ) * V_Phi_Rei_squ_p_plus_1_vec(kk, iiuav) ...
                                                                    * ( ( sech( ( gamma0 / 2 ) * V_Phi_Rei_div_pi_vec(kk, iiuav) ) ...
                                                                    / tanh( ( gamma0 / 2 ) * V_Phi_Rei_div_pi_vec(kk, iiuav) ) ) ^ 2 ) * wei_vec(kk, iiuav);
        else
            Phi_bar_psi_e_node_2(kk, 1) = 2 * beta_Phi_1 * ( ( abs( V_Phi_Rei_div_pi_vec(kk, iiuav) ) ) ^ 2 ) * wei_vec(kk, iiuav) ...
                                                                    + ( 2 * pp0 + 1 ) * beta_Phi_2 * V_Phi_Rei_squ_2p_vec(kk, iiuav) * wei_vec(kk, iiuav);
        end
    end
end

== matlab function sim_new_traj_only_att_ctrl/combine tau1 ==
  data: dw_1 input; dw_vec output; dw_2 input; dw_3 input; dw_4 input; dw_5 input
function dw_vec = fcn(dw_1, dw_2, dw_3, dw_4, dw_5)
%%%% 合并辅助姿态角速率
dw_vec = [dw_1(:), dw_2(:), dw_3(:), dw_4(:), dw_5(:)];

== matlab function sim_new_traj_only_att_ctrl/combine theta_Si_beta_w_1 ==
  data: theta_Si_beta_w_1_node_1 input; theta_Si_beta_w_1_node_2 input; theta_Si_beta_w_1_node_3 input; theta_Si_beta_w_1_node_4 input; theta_Si_beta_w_1_node_5 input; theta_Si_beta_w_1_vec output
function theta_Si_beta_w_1_vec  = fcn(theta_Si_beta_w_1_node_1, theta_Si_beta_w_1_node_2, theta_Si_beta_w_1_node_3, ...
                                                                        theta_Si_beta_w_1_node_4, theta_Si_beta_w_1_node_5)
%%%% 合并误差非线性项
theta_Si_beta_w_1_vec = zeros(3,5);
theta_Si_beta_w_1_vec(:,1) = theta_Si_beta_w_1_node_1(:);
theta_Si_beta_w_1_vec(:,2) = theta_Si_beta_w_1_node_2(:);
theta_Si_beta_w_1_vec(:,3) = theta_Si_beta_w_1_node_3(:);
theta_Si_beta_w_1_vec(:,4) = theta_Si_beta_w_1_node_4(:);
theta_Si_beta_w_1_vec(:,5) = theta_Si_beta_w_1_node_5(:);

== matlab function sim_new_traj_only_att_ctrl/combine theta_Si_beta_w_2 ==
  data: theta_Si_beta_w_2_node_1 input; theta_Si_beta_w_2_node_2 input; theta_Si_beta_w_2_node_3 input; theta_Si_beta_w_2_node_4 input; theta_Si_beta_w_2_node_5 input; theta_Si_beta_w_2_vec output
function theta_Si_beta_w_2_vec  = fcn(theta_Si_beta_w_2_node_1, theta_Si_beta_w_2_node_2, theta_Si_beta_w_2_node_3, ...
                                                                        theta_Si_beta_w_2_node_4, theta_Si_beta_w_2_node_5)
%%%% 合并误差非线性项
theta_Si_beta_w_2_vec = zeros(3,5);
theta_Si_beta_w_2_vec(:,1) = theta_Si_beta_w_2_node_1(:);
theta_Si_beta_w_2_vec(:,2) = theta_Si_beta_w_2_node_2(:);
theta_Si_beta_w_2_vec(:,3) = theta_Si_beta_w_2_node_3(:);
theta_Si_beta_w_2_vec(:,4) = theta_Si_beta_w_2_node_4(:);
theta_Si_beta_w_2_vec(:,5) = theta_Si_beta_w_2_node_5(:);

== matlab function sim_new_traj_only_att_ctrl/combine theta_sigma_bar_w_tilt ==
  data: theta_sigma_bar_w_tilt_1_1 input; theta_sigma_bar_w_tilt_1_2 input; theta_sigma_bar_w_tilt_1_3 input; theta_sigma_bar_w_tilt_1_4 input; theta_sigma_bar_w_tilt_1_5 input; theta_sigma_bar_w_tilt_1_vec output; theta_sigma_bar_w_tilt_2_1 input; theta_sigma_bar_w_tilt_2_vec output; theta_sigma_bar_w_tilt_2_2 input; theta_sigma_bar_w_tilt_2_3 input; theta_sigma_bar_w_tilt_2_4 input; theta_sigma_bar_w_tilt_2_5 input
function [theta_sigma_bar_w_tilt_1_vec, theta_sigma_bar_w_tilt_2_vec]  = fcn(theta_sigma_bar_w_tilt_1_1, theta_sigma_bar_w_tilt_1_2, theta_sigma_bar_w_tilt_1_3, theta_sigma_bar_w_tilt_1_4, theta_sigma_bar_w_tilt_1_5, ...
                                                                                                                                            theta_sigma_bar_w_tilt_2_1, theta_sigma_bar_w_tilt_2_2, theta_sigma_bar_w_tilt_2_3, theta_sigma_bar_w_tilt_2_4, theta_sigma_bar_w_tilt_2_5)
%%%% 合并领导者位置观测器输出结果
theta_sigma_bar_w_tilt_1_vec = [theta_sigma_bar_w_tilt_1_1(:), theta_sigma_bar_w_tilt_1_2(:), theta_sigma_bar_w_tilt_1_3(:), theta_sigma_bar_w_tilt_1_4(:), theta_sigma_bar_w_tilt_1_5(:)];
theta_sigma_bar_w_tilt_2_vec = [theta_sigma_bar_w_tilt_2_1(:), theta_sigma_bar_w_tilt_2_2(:), theta_sigma_bar_w_tilt_2_3(:), theta_sigma_bar_w_tilt_2_4(:), theta_sigma_bar_w_tilt_2_5(:)];

== matlab function sim_new_traj_only_att_ctrl/combine wci dwci ==
  data: wci_node_1 input; wci_vec output; wci_node_2 input; wci_node_3 input; wci_node_4 input; wci_node_5 input; dwci_vec output; dwci_node_1 input; dwci_node_2 input; dwci_node_3 input; dwci_node_4 input; dwci_node_5 input
function [wci_vec, dwci_vec] = fcn(wci_node_1, wci_node_2, wci_node_3, wci_node_4, wci_node_5, ...
                                                                dwci_node_1, dwci_node_2, dwci_node_3, dwci_node_4, dwci_node_5)
%%%% 合并姿态角速率指令及其导数
wci_vec = [wci_node_1(:), wci_node_2(:), wci_node_3(:), wci_node_4(:), wci_node_5(:)];
dwci_vec = [dwci_node_1(:), dwci_node_2(:), dwci_node_3(:), dwci_node_4(:), dwci_node_5(:)];

== matlab function sim_new_traj_only_att_ctrl/combine wei Qei Rei ==
  data: wei_1 input; wei_vec output; wei_2 input; wei_3 input; wei_4 input; wei_5 input; Qei_1 input; Qei_2 input; Qei_3 input; Qei_4 input; Qei_5 input; Rei_1 input; Rei_2 input; Rei_3 input; Rei_4 input; Rei_5 input; Qei_vec output; Rei_vec output
function [wei_vec, Qei_vec, Rei_vec] = fcn(wei_1, wei_2, wei_3, wei_4, wei_5, ...
                                                                            Qei_1, Qei_2, Qei_3, Qei_4, Qei_5, ...
                                                                            Rei_1, Rei_2, Rei_3, Rei_4, Rei_5)
%%%% 合并姿态角速率误差/四元数误差/姿态旋转矩阵误差
wei_vec = zeros(3,5);
wei_vec(:,1) = wei_1(:);
wei_vec(:,2) = wei_2(:);
wei_vec(:,3) = wei_3(:);
wei_vec(:,4) = wei_4(:);
wei_vec(:,5) = wei_5(:);

Qei_vec = zeros(4,5);
Qei_vec(:,1) = Qei_1(:);
Qei_vec(:,2) = Qei_2(:);
Qei_vec(:,3) = Qei_3(:);
Qei_vec(:,4) = Qei_4(:);
Qei_vec(:,5) = Qei_5(:);

Rei_vec = zeros(3,3,5);
Rei_vec(:,:,1) = Rei_1;
Rei_vec(:,:,2) = Rei_2;
Rei_vec(:,:,3) = Rei_3;
Rei_vec(:,:,4) = Rei_4;
Rei_vec(:,:,5) = Rei_5;

== matlab function sim_new_traj_only_att_ctrl/generate angular rate disturbance agent 1 ==
  data: dw_1 output; dw_aa_t input; dw_ff_t input; dw_phi_t input; t input
function dw_1 = fcn(dw_aa_t, dw_ff_t, dw_phi_t, t)
%%%% 姿态动力学方程中的扰动项设置
epsil_t = zeros(3, 1);

for kk = 1:5
    epsil_t = epsil_t + dw_aa_t(:, kk) .* sin( 2 * pi * dw_ff_t(:, kk) * t + dw_phi_t(:, kk) );
end

dw_1 = [ epsil_t(1) + 1.6 * sin( 0.4 * t ) + 2.0 * cos( 0.5 * t ) + 1.4 * sin( 0.7 * t ) ...
                + 4 * exp( -0.1 * t ) * sin( 0.8 * t ) + 3 / ( 1 + exp( -0.2 * ( t - 15 ) ) ); ...
                epsil_t(2) + 1.2 * sin( 0.2 * t ) + 3 * cos( 0.4 * t ) + 0.8 * sin( 0.6 * t ) ...
                + 2 * exp( -0.15 * t ) * cos( 1.2 * t ) + 3 / ( 1 + exp( -0.3 * ( t - 25 ) ) ); ...
                epsil_t(3) + 1.8 * sin( 0.2 * t ) + 1.6 * sin( 0.3 * t ) + 1.6 * cos( 0.4 * t ) ...
                + 4 * exp( -0.05 * t ) * sin( 0.5 * t + pi / 4 ) + 3 / ( 1 + exp( -0.5 * ( t - 20 ) ) ) ];

== matlab function sim_new_traj_only_att_ctrl/generate angular rate disturbance agent 2 ==
  data: dw_2 output; dw_aa_t input; dw_ff_t input; dw_phi_t input; t input
function dw_2 = fcn(dw_aa_t, dw_ff_t, dw_phi_t, t)
%%%% 姿态动力学方程中的扰动项设置
epsil_t = zeros(3, 1);

for kk = 1:5
    epsil_t = epsil_t + dw_aa_t(:, kk) .* sin( 2 * pi * dw_ff_t(:, kk) * t + dw_phi_t(:, kk) );
end

dw_2 = [ epsil_t(1) + 1.6 * sin( 0.2 * t ) + 2.0 * cos( 0.3 * t ) + 1.4 * sin( 0.5 * t ) ...
                + 4 * exp( -0.1 * t ) * sin( 0.5 * t ) + 3 / ( 1 + exp( -0.2 * ( t - 15 ) ) ); ...
                epsil_t(2) + 1.2 * sin( 0.1 * t ) + 3 * cos( 0.2 * t ) + 0.8 * sin( 0.4 * t ) ...
                + 2 * exp( -0.15 * t ) * cos( 0.6 * t ) + 3 / ( 1 + exp( -0.3 * ( t - 25 ) ) ); ...
                epsil_t(3) + 1.8 * sin( 0.1 * t ) + 1.6 * sin( 0.2 * t ) + 1.6 * cos( 0.3 * t ) ...
                + 4 * exp( -0.05 * t ) * sin( 0.4 * t + pi / 4 ) + 3 / ( 1 + exp( -0.5 * ( t - 20 ) ) ) ];

== matlab function sim_new_traj_only_att_ctrl/generate angular rate disturbance agent 3 ==
  data: dw_3 output; dw_aa_t input; dw_ff_t input; dw_phi_t input; t input
function dw_3 = fcn(dw_aa_t, dw_ff_t, dw_phi_t, t)
%%%% 姿态动力学方程中的扰动项设置
epsil_t = zeros(3, 1);

for kk = 1:5
    epsil_t = epsil_t + dw_aa_t(:, kk) .* sin( 2 * pi * dw_ff_t(:, kk) * t + dw_phi_t(:, kk) );
end

dw_3 = [ epsil_t(1) + 1.6 * sin( 0.2 * t ) + 2.0 * cos( 0.3 * t ) + 1.4 * sin( 0.5 * t ) ...
                + 4 * exp( -0.1 * t ) * sin( 0.5 * t ) + 3 / ( 1 + exp( -0.2 * ( t - 15 ) ) ); ...
                epsil_t(2) + 1.2 * sin( 0.1 * t ) + 3 * cos( 0.2 * t ) + 0.8 * sin( 0.4 * t ) ...
                + 2 * exp( -0.15 * t ) * cos( 0.6 * t ) + 3 / ( 1 + exp( -0.3 * ( t - 25 ) ) ); ...
                epsil_t(3) + 1.8 * sin( 0.1 * t ) + 1.6 * sin( 0.2 * t ) + 1.6 * cos( 0.3 * t ) ...
                + 4 * exp( -0.05 * t ) * sin( 0.4 * t + pi / 4 ) + 3 / ( 1 + exp( -0.5 * ( t - 20 ) ) ) ];

== matlab function sim_new_traj_only_att_ctrl/generate angular rate disturbance agent 4 ==
  data: dw_4 output; dw_aa_t input; dw_ff_t input; dw_phi_t input; t input
function dw_4 = fcn(dw_aa_t, dw_ff_t, dw_phi_t, t)
%%%% 姿态动力学方程中的扰动项设置
epsil_t = zeros(3, 1);

for kk = 1:5
    epsil_t = epsil_t + dw_aa_t(:, kk) .* sin( 2 * pi * dw_ff_t(:, kk) * t + dw_phi_t(:, kk) );
end

dw_4 = [ epsil_t(1) + 1.6 * sin( 0.2 * t ) + 2.0 * cos( 0.3 * t ) + 1.4 * sin( 0.5 * t ) ...
                + 4 * exp( -0.1 * t ) * sin( 0.5 * t ) + 3 / ( 1 + exp( -0.2 * ( t - 15 ) ) ); ...
                epsil_t(2) + 1.2 * sin( 0.1 * t ) + 3 * cos( 0.2 * t ) + 0.8 * sin( 0.4 * t ) ...
                + 2 * exp( -0.15 * t ) * cos( 0.6 * t ) + 3 / ( 1 + exp( -0.3 * ( t - 25 ) ) ); ...
                epsil_t(3) + 1.8 * sin( 0.1 * t ) + 1.6 * sin( 0.2 * t ) + 1.6 * cos( 0.3 * t ) ...
                + 4 * exp( -0.05 * t ) * sin( 0.4 * t + pi / 4 ) + 3 / ( 1 + exp( -0.5 * ( t - 20 ) ) ) ];

== matlab function sim_new_traj_only_att_ctrl/generate angular rate disturbance agent 5 ==
  data: dw_5 output; dw_aa_t input; dw_ff_t input; dw_phi_t input; t input
function dw_5 = fcn(dw_aa_t, dw_ff_t, dw_phi_t, t)
%%%% 姿态动力学方程中的扰动项设置
epsil_t = zeros(3, 1);

for kk = 1:5
    epsil_t = epsil_t + dw_aa_t(:, kk) .* sin( 2 * pi * dw_ff_t(:, kk) * t + dw_phi_t(:, kk) );
end

dw_5 = [ epsil_t(1) + 1.6 * sin( 0.2 * t ) + 2.0 * cos( 0.3 * t ) + 1.4 * sin( 0.5 * t ) ...
                + 4 * exp( -0.1 * t ) * sin( 0.5 * t ) + 3 / ( 1 + exp( -0.2 * ( t - 15 ) ) ); ...
                epsil_t(2) + 1.2 * sin( 0.1 * t ) + 3 * cos( 0.2 * t ) + 0.8 * sin( 0.4 * t ) ...
                + 2 * exp( -0.15 * t ) * cos( 0.6 * t ) + 3 / ( 1 + exp( -0.3 * ( t - 25 ) ) ); ...
                epsil_t(3) + 1.8 * sin( 0.1 * t ) + 1.6 * sin( 0.2 * t ) + 1.6 * cos( 0.3 * t ) ...
                + 4 * exp( -0.05 * t ) * sin( 0.4 * t + pi / 4 ) + 3 / ( 1 + exp( -0.5 * ( t - 20 ) ) ) ];

== matlab function sim_new_traj_only_att_ctrl/trans to column100 ==
  data: x input; y output
function y = fcn(x)
y = x(:);

== matlab function sim_new_traj_only_att_ctrl/trans to column101 ==
  data: x input; y output
function y = fcn(x)
y = x(:);

== matlab function sim_new_traj_only_att_ctrl/trans to column102 ==
  data: x input; y output
function y = fcn(x)
y = x(:);

== matlab function sim_new_traj_only_att_ctrl/trans to column103 ==
  data: x input; y output
function y = fcn(x)
y = x(:);

== matlab function sim_new_traj_only_att_ctrl/trans to column104 ==
  data: x input; y output
function y = fcn(x)
y = x(:);

== matlab function sim_new_traj_only_att_ctrl/trans to column105 ==
  data: x input; y output
function y = fcn(x)
y = x(:);

== matlab function sim_new_traj_only_att_ctrl/cal Phi_bar_psi_e agent 3 ==
  data: pp0 input; Phi_bar_psi_e_node_3 output; beta_Phi_1 input; beta_Phi_2 input; thr_p_plus_1 input; gamma0 input; eps_s_bar_div_pi input; wei_vec input; S_bar_vec input; V_Phi_Rei_div_pi_vec input; V_Phi_Rei_squ_p_min_1_vec input; V_Phi_Rei_squ_p_plus_1_vec input; V_Phi_Rei_squ_2p_vec input
function Phi_bar_psi_e_node_3 = fcn(pp0, beta_Phi_1, beta_Phi_2, thr_p_plus_1, gamma0, ...
                                                                    eps_s_bar_div_pi, wei_vec, S_bar_vec, V_Phi_Rei_div_pi_vec, ...
                                                                    V_Phi_Rei_squ_p_min_1_vec, V_Phi_Rei_squ_p_plus_1_vec, V_Phi_Rei_squ_2p_vec)
%%%% 计算姿态误差项
iiuav = 3;
Phi_bar_psi_e_node_3 = zeros(3,1);
for kk = 1:3
    if S_bar_vec(kk, iiuav) == 0
        Phi_bar_psi_e_node_3(kk, 1) = thr_p_plus_1 * ( pp0 + 1 ) * V_Phi_Rei_div_pi_vec(kk, iiuav) ...
                                                                * V_Phi_Rei_squ_p_min_1_vec(kk, iiuav) * wei_vec(kk, iiuav) ...
                                                                / ( 2 * tanh( ( gamma0 / 2 ) * V_Phi_Rei_div_pi_vec(kk, iiuav) ) ) ...
                                                                + ( thr_p_plus_1 * gamma0 / 4 ) * V_Phi_Rei_squ_p_plus_1_vec(kk, iiuav) ...
                                                                * ( ( sech( ( gamma0 / 2 ) * V_Phi_Rei_div_pi_vec(kk, iiuav) ) ...
                                                                / tanh( ( gamma0 / 2 ) * V_Phi_Rei_div_pi_vec(kk, iiuav) ) ) ^ 2 ) * wei_vec(kk, iiuav);
    else
        if abs( V_Phi_Rei_div_pi_vec ) > eps_s_bar_div_pi
            Phi_bar_psi_e_node_3(kk, 1) = thr_p_plus_1 * ( pp0 + 1 ) * V_Phi_Rei_div_pi_vec(kk, iiuav) ...
                                                                    * V_Phi_Rei_squ_p_min_1_vec(kk, iiuav) * wei_vec(kk, iiuav) ...
                                                                    / ( 2 * tanh( ( gamma0 / 2 ) * V_Phi_Rei_div_pi_vec(kk, iiuav) ) ) ...
                                                                    + ( thr_p_plus_1 * gamma0 / 4 ) * V_Phi_Rei_squ_p_plus_1_vec(kk, iiuav) ...
                                                                    * ( ( sech( ( gamma0 / 2 ) * V_Phi_Rei_div_pi_vec(kk, iiuav) ) ...
                                                                    / tanh( ( gamma0 / 2 ) * V_Phi_Rei_div_pi_vec(kk, iiuav) ) ) ^ 2 ) * wei_vec(kk, iiuav);
        else
            Phi_bar_psi_e_node_3(kk, 1) = 2 * beta_Phi_1 * ( ( abs( V_Phi_Rei_div_pi_vec(kk, iiuav) ) ) ^ 2 ) * wei_vec(kk, iiuav) ...
                                                                    + ( 2 * pp0 + 1 ) * beta_Phi_2 * V_Phi_Rei_squ_2p_vec(kk, iiuav) * wei_vec(kk, iiuav);
        end
    end
end

== matlab function sim_new_traj_only_att_ctrl/trans to column106 ==
  data: x input; y output
function y = fcn(x)
y = x(:);

== matlab function sim_new_traj_only_att_ctrl/trans to column107 ==
  data: x input; y output
function y = fcn(x)
y = x(:);

== matlab function sim_new_traj_only_att_ctrl/trans to column108 ==
  data: x input; y output
function y = fcn(x)
y = x(:);

== matlab function sim_new_traj_only_att_ctrl/trans to column109 ==
  data: x input; y output
function y = fcn(x)
y = x(:);

== matlab function sim_new_traj_only_att_ctrl/trans to column110 ==
  data: x input; y output
function y = fcn(x)
y = x(:);

== matlab function sim_new_traj_only_att_ctrl/trans to column111 ==
  data: x input; y output
function y = fcn(x)
y = x(:);

== matlab function sim_new_traj_only_att_ctrl/trans to column112 ==
  data: x input; y output
function y = fcn(x)
y = x(:);

== matlab function sim_new_traj_only_att_ctrl/trans to column113 ==
  data: x input; y output
function y = fcn(x)
y = x(:);

== matlab function sim_new_traj_only_att_ctrl/trans to column114 ==
  data: x input; y output
function y = fcn(x)
y = x(:);

== matlab function sim_new_traj_only_att_ctrl/trans to column115 ==
  data: x input; y output
function y = fcn(x)
y = x(:);

== matlab function sim_new_traj_only_att_ctrl/trans to column116 ==
  data: x input; y output
function y = fcn(x)
y = x(:);

== matlab function sim_new_traj_only_att_ctrl/trans to column117 ==
  data: x input; y output
function y = fcn(x)
y = x(:);

== matlab function sim_new_traj_only_att_ctrl/trans to column118 ==
  data: x input; y output
function y = fcn(x)
y = x(:);

== matlab function sim_new_traj_only_att_ctrl/trans to column119 ==
  data: x input; y output
function y = fcn(x)
y = x(:);

== matlab function sim_new_traj_only_att_ctrl/trans to column120 ==
  data: x input; y output
function y = fcn(x)
y = x(:);

== matlab function sim_new_traj_only_att_ctrl/trans to column121 ==
  data: x input; y output
function y = fcn(x)
y = x(:);

== matlab function sim_new_traj_only_att_ctrl/trans to column122 ==
  data: x input; y output
function y = fcn(x)
y = x(:);

== matlab function sim_new_traj_only_att_ctrl/trans to column123 ==
  data: x input; y output
function y = fcn(x)
y = x(:);

== matlab function sim_new_traj_only_att_ctrl/trans to column124 ==
  data: x input; y output
function y = fcn(x)
y = x(:);

== matlab function sim_new_traj_only_att_ctrl/trans to column125 ==
  data: x input; y output
function y = fcn(x)
y = x(:);

== matlab function sim_new_traj_only_att_ctrl/trans to column61 ==
  data: x input; y output
function y = fcn(x)
y = x(:);
